simulink model "HybridModel1"  (R2020a)
settings: Solver=FixedStepAuto  StartTime=0  StopTime=10.67  FixedStep=0.01  RelTol=1e-3
libraries: simulink x1, cstblocks x1
settings Model: Creator=Brock  LastModifiedBy=Brock

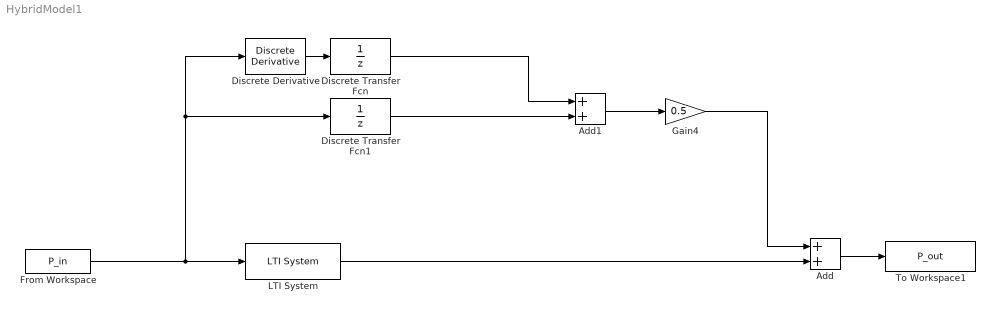
== system HybridModel1 ==
  Add : Sum
  Add1 : Sum
  Discrete Transfer Fcn : DiscreteTransferFcn  Denominator=[1 0]  SampleTime=0.1
  Discrete Transfer Fcn1 : DiscreteTransferFcn  Denominator=[1 0]  SampleTime=0.1
  Discrete Derivative : simulink/Discrete/Discrete Derivative  gainval=VSA  ICPrevScaledInput=0.0  OutMin=[]  OutMax=[]  OutDataType=fixdt(1, 16)  OutScaling=2^-10  DoSatur=off
  From Workspace : FromWorkspace  VariableName=P_in
  Gain4 : Gain  Gain=0.5
  LTI System : cstblocks/LTI System  sys=TF_sm  IC=[]
  To Workspace1 : ToWorkspace  VariableName=P_out  SampleTime=-1
  wires:
  From Workspace/1 -> Discrete Transfer Fcn1/1, Discrete Derivative/1, LTI System/1
  Add/1 -> To Workspace1/1
  LTI System/1 -> Add/2
  Gain4/1 -> Add/1
  Discrete Transfer Fcn/1 -> Add1/1
  Discrete Derivative/1 -> Discrete Transfer Fcn/1
  Add1/1 -> Gain4/1
  Discrete Transfer Fcn1/1 -> Add1/2
